simulink model "Copy_of_Model_vmaRHTS_R2019b"  (R2023a)
settings: Solver=ode4  StartTime=0.0  StopTime=tend  FixedStep=dt  RelTol=1e-3
undefined symbols (not defined in the file or in its folder): a0, a1, a2, a3, a4, a5, a6, a7, A_cplant, Ag, AgN, alpha1, alpha2, B_cplant, C_cplant, C_phys_5dof, CNrt, Continuous, CRrt, D_cplant, dt, dv1, dv2, EQ_intensity, EQ_sw, F, FN, K, K_1, K_2, K_phys_5dof, Kbar_inv, KI, KI_1, KI_2, KNbar_inv, Koo, Kot, l, lN, M_phys_5dof, MNrt, MRrt, Rbar, RNbar, Seed_snr, Time
libraries: simulink x6, slpidlib x4, ctrlSharedLib x3, sldrtlib x1
(part 1 of 3)
settings Model: Creator=icu327  LastModifiedBy=liangyu
settings SolverCC: AlgebraicLoopSolver=TrustRegion
settings DataIOCC: SaveFormat=Array  ReturnWorkspaceOutputs=off
settings DebuggingCC: UnconnectedInputMsg=warning  UnconnectedOutputMsg=warning  UnconnectedLineMsg=warning  ArithmeticOperatorsInVariantConditions=warning
settings HardwareCC: ProdBitPerLong=64  ProdHWDeviceType=Intel->x86-64 (Linux 64)
settings ModelReferenceCC: EnableRefExpFcnMdlSchedulingChecks=on
settings SFSimCC: CustomCodeUndefinedFunction=UseInterfaceOnly
settings RTWCC: Description=Simulink Desktop Real-Time  SystemTargetFile=sldrt.tlc  TemplateMakefile=sldrt.tmf  RTWCompilerOptimization=on
settings CodeAppCC: MaxIdLength=95  StateflowObjectComments=on
settings SimulinkDesktopRealTimeCC: TargetLibSuffix=_sldrt.a  TargetPreCompLibLocation=C:\Program Files\MATLAB\R2023a\toolbox\sldrt\lib\win64

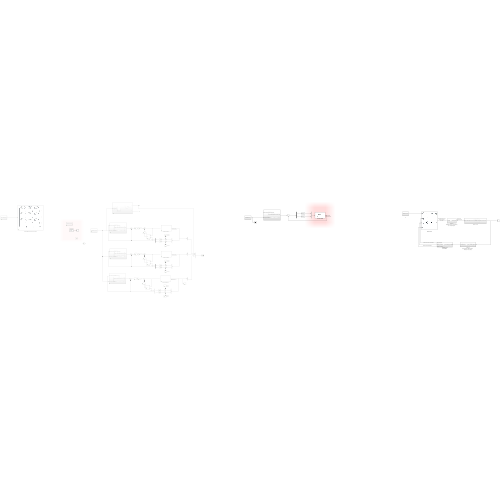
[thumbnail: Simulink's stored preview of the top-level diagram]
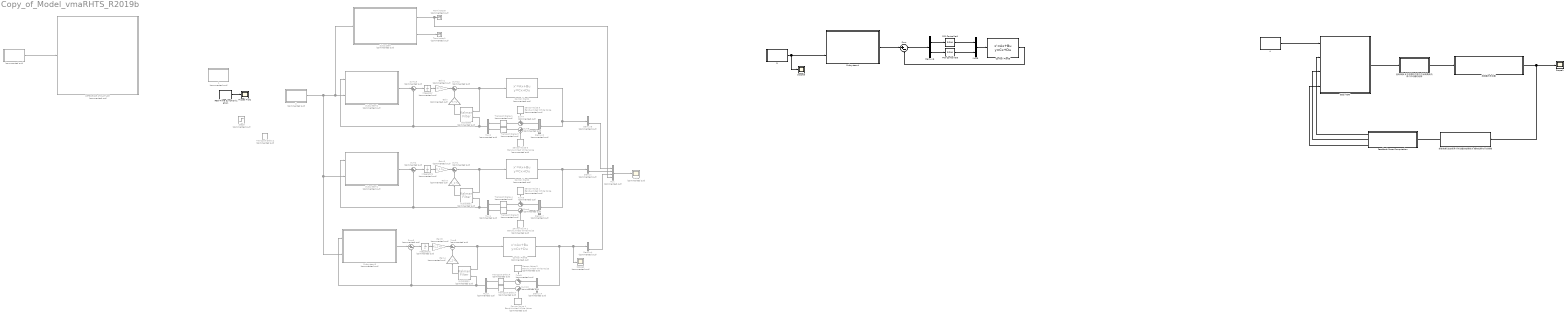
== system Copy_of_Model_vmaRHTS_R2019b ==
  " " : Subsystem  Commented=on
  " 1" : Subsystem  Commented=on
  " 2" : Subsystem  Commented=on
  " 3" : Subsystem
  " 4" : Subsystem
  " REFERENCE STRUCTURE" : Subsystem  Commented=on
      mask Display: image('$imagefile'); % Use "Edit Image" on toolstrip to change.
  " 数值子结构" : Subsystem
      mask Display: image('$imagefile'); % Use "Edit Image" on toolstrip to change.
  Control Plant1 : StateSpace  Commented=on  A=A_cplant  B=B_cplant  C=C_cplant  D=D_cplant  InitialCondition=0
  Control Plant2 : StateSpace  Commented=on  A=A_cplant  B=B_cplant  C=C_cplant  D=D_cplant  InitialCondition=0
  Control Plant3 : StateSpace  Commented=on  A=A_cplant  B=B_cplant  C=C_cplant  D=D_cplant  InitialCondition=0
  Control Plant5 : StateSpace  A=A_cplant  B=B_cplant  C=C_cplant  D=D_cplant  InitialCondition=0
  Demux{,1..5} (6 alike) : Demux  Commented=on  Outputs=2
  Demux6 : Demux  Outputs=2
  Feedback Force Computation : Subsystem
  Gain : Gain  Commented=on  Gain=K  Multiplication=Matrix(K*u) (u vector)
  Gain1 : Gain  Commented=on  Gain=KI  Multiplication=Matrix(K*u) (u vector)
  Gain2 : Gain  Commented=on  Gain=K_1  Multiplication=Matrix(K*u) (u vector)
  Gain3 : Gain  Commented=on  Gain=KI_1  Multiplication=Matrix(K*u) (u vector)
  Gain4 : Gain  Commented=on  Gain=K_2  Multiplication=Matrix(K*u) (u vector)
  Gain5 : Gain  Commented=on  Gain=KI_2  Multiplication=Matrix(K*u) (u vector)
  Integrator : Integrator  Commented=on
  Integrator1 : Integrator  Commented=on
  Integrator2 : Integrator  Commented=on
  Missed Ticks : Scope
  Mux : Mux  Commented=on
  Mux1 : Mux  Commented=on  Inputs=2
  Mux2 : Mux  Commented=on  Inputs=2
  Mux3 : Mux  Commented=on  Inputs=2
  Mux5 : Mux  Inputs=2
  PID Controller1 : slpidlib/PID Controller  Controller=PID  Form=Parallel  TimeDomain=Discrete-time  UseExternalTs=off  SampleTime=-1  IntegratorMethod=Forward Euler  FilterMethod=Forward Euler  ControllerParametersSource=internal  P=1  I=50  UseKiTs=off  D=1e-10  N=100  UseFilter=off  TunerSelectOption=Transfer Function Based (PID Tuner App)  InitialConditionSource=internal  InitialConditionForIntegrator=0  InitialConditionForFilter=0  DifferentiatorICPrevScaledInput=0  ExternalReset=none  TrackingMode=off  Kt=1  LimitOutput=off  SatLimitsSource=internal  UpperSaturationLimit=inf  LowerSaturationLimit=-inf  LinearizeAsGain=on  AntiWindupMode=none  Kb=1  LimitIntegrator=off  UpperIntegratorSaturationLimit=inf  LowerIntegratorSaturationLimit=-inf  POutMin=[]  POutMax=[]  IOutMin=[]  IOutMax=[]  DOutMin=[]  DOutMax=[]  NOutMin=[]  NOutMax=[]  SumOutMin=[]  SumOutMax=[]  SaturationOutMin=[]  SaturationOutMax=[]  PParamMin=[]  PParamMax=[]  IParamMin=[]  IParamMax=[]  DParamMin=[]  DParamMax=[]  NParamMin=[]  NParamMax=[]  KbParamMin=[]  KbParamMax=[]  KtParamMin=[]  KtParamMax=[]  KbOutMin=[]  KbOutMax=[]  KtOutMin=[]  KtOutMax=[]  IntegratorOutMin=[]  IntegratorOutMax=[]  FilterOutMin=[]  FilterOutMax=[]  SumI1OutMin=[]  SumI1OutMax=[]  SumI2OutMin=[]  SumI2OutMax=[]  SumI3OutMin=[]  SumI3OutMax=[]  SumI4OutMin=[]  SumI4OutMax=[]  SumDOutMin=[]  SumDOutMax=[]  DifferentiatorOutMin=[]  DifferentiatorOutMax=[]  FilterDiffOutCoefMin=[]  FilterDiffOutCoefMax=[]  ReciprocalOutMin=[]  ReciprocalOutMax=[]  SumDenOutMin=[]  SumDenOutMax=[]  SumNumOutMin=[]  SumNumOutMax=[]  DivideOutMin=[]  DivideOutMax=[]  UdiffTsProdOutMin=[]  UdiffTsProdOutMax=[]  NTsProdOutMin=[]  NTsProdOutMax=[]  UintegralTsProdOutMin=[]  UintegralTsProdOutMax=[]  UngainTsProdOutMin=[]  UngainTsProdOutMax=[]  ClampingZeroOutDataTypeStr=Inherit: Inherit via back propagation  ClampingZeroOutMin=[]  ClampingZeroOutMax=[]  FilterDenConstantOutDataTypeStr=Inherit: Inherit via back propagation  FilterDenConstantOutMin=[]  FilterDenConstantOutMax=[]  PCopyOutDataTypeStr=Inherit: Inherit via back propagation  PCopyOutMin=[]  PCopyOutMax=[]  NCopyOutDataTypeStr=Inherit: Inherit via back propagation  NCopyOutMin=[]  NCopyOutMax=[]  IntegratorContinuousStateAttributes=''  IntegratorStateMustResolveToSignalObject=off  IntegratorRTWStateStorageClass=Auto  FilterContinuousStateAttributes=''  FilterStateMustResolveToSignalObject=off  FilterRTWStateStorageClass=Auto  ParallelPVariant=InternalParameters  IdealPVariant=Disabled  IVariant=InternalParameters  DVariant=InternalParameters  IntegratorVariant=Discrete  SatVariant=Disabled  AWVariant=Passthrough  PCopyVariant=Disabled  TRVariant=Disabled  FdbkBlocksVariant=Forward  IdealPFdbkVariant=Disabled  SatFdbkVariant=Disabled  DerivativeFilterVariant=Differentiator  NVariant=Passthrough  NCopyVariant=Disabled_SignalSpec  FilterICVariant=InternalICsDifferentiator  IntegratorICVariant=InternalICs  ExternalResetVariant=Disabled  TRSumVariant=Passthrough  SumFdbkVariant=Disabled  SumVariant=Sum_PID  TsampFilterVariant=InternalTs  TsampNgainVariant=Passthrough  TsampIntegralVariant=Disabled_SignalSpec  ExternalSaturationOutDataTypeStr=Inherit: Same as second input
  PID Controller3 : slpidlib/PID Controller  Controller=PID  Form=Parallel  TimeDomain=Discrete-time  UseExternalTs=off  SampleTime=-1  IntegratorMethod=Forward Euler  FilterMethod=Forward Euler  ControllerParametersSource=internal  P=1  I=50  UseKiTs=off  D=1e-10  N=100  UseFilter=on  TunerSelectOption=Transfer Function Based (PID Tuner App)  InitialConditionSource=internal  InitialConditionForIntegrator=0  InitialConditionForFilter=0  DifferentiatorICPrevScaledInput=0  ExternalReset=none  TrackingMode=off  Kt=1  LimitOutput=off  SatLimitsSource=internal  UpperSaturationLimit=inf  LowerSaturationLimit=-inf  LinearizeAsGain=on  AntiWindupMode=none  Kb=1  LimitIntegrator=off  UpperIntegratorSaturationLimit=inf  LowerIntegratorSaturationLimit=-inf  POutMin=[]  POutMax=[]  IOutMin=[]  IOutMax=[]  DOutMin=[]  DOutMax=[]  NOutMin=[]  NOutMax=[]  SumOutMin=[]  SumOutMax=[]  SaturationOutMin=[]  SaturationOutMax=[]  PParamMin=[]  PParamMax=[]  IParamMin=[]  IParamMax=[]  DParamMin=[]  DParamMax=[]  NParamMin=[]  NParamMax=[]  KbParamMin=[]  KbParamMax=[]  KtParamMin=[]  KtParamMax=[]  KbOutMin=[]  KbOutMax=[]  KtOutMin=[]  KtOutMax=[]  IntegratorOutMin=[]  IntegratorOutMax=[]  FilterOutMin=[]  FilterOutMax=[]  SumI1OutMin=[]  SumI1OutMax=[]  SumI2OutMin=[]  SumI2OutMax=[]  SumI3OutMin=[]  SumI3OutMax=[]  SumI4OutMin=[]  SumI4OutMax=[]  SumDOutMin=[]  SumDOutMax=[]  DifferentiatorOutMin=[]  DifferentiatorOutMax=[]  FilterDiffOutCoefMin=[]  FilterDiffOutCoefMax=[]  ReciprocalOutMin=[]  ReciprocalOutMax=[]  SumDenOutMin=[]  SumDenOutMax=[]  SumNumOutMin=[]  SumNumOutMax=[]  DivideOutMin=[]  DivideOutMax=[]  UdiffTsProdOutMin=[]  UdiffTsProdOutMax=[]  NTsProdOutMin=[]  NTsProdOutMax=[]  UintegralTsProdOutMin=[]  UintegralTsProdOutMax=[]  UngainTsProdOutMin=[]  UngainTsProdOutMax=[]  ClampingZeroOutDataTypeStr=Inherit: Inherit via back propagation  ClampingZeroOutMin=[]  ClampingZeroOutMax=[]  FilterDenConstantOutDataTypeStr=Inherit: Inherit via back propagation  FilterDenConstantOutMin=[]  FilterDenConstantOutMax=[]  PCopyOutDataTypeStr=Inherit: Inherit via back propagation  PCopyOutMin=[]  PCopyOutMax=[]  NCopyOutDataTypeStr=Inherit: Inherit via back propagation  NCopyOutMin=[]  NCopyOutMax=[]  IntegratorContinuousStateAttributes=''  IntegratorStateMustResolveToSignalObject=off  IntegratorRTWStateStorageClass=Auto  FilterContinuousStateAttributes=''  FilterStateMustResolveToSignalObject=off  FilterRTWStateStorageClass=Auto  ParallelPVariant=InternalParameters  IdealPVariant=Disabled  IVariant=InternalParameters  DVariant=InternalParameters  IntegratorVariant=Discrete  SatVariant=Disabled  AWVariant=Passthrough  PCopyVariant=Disabled  TRVariant=Disabled  FdbkBlocksVariant=Forward  IdealPFdbkVariant=Disabled  SatFdbkVariant=Disabled  DerivativeFilterVariant=ForwardEulerFilter  NVariant=InternalParameters  NCopyVariant=Disabled  FilterICVariant=InternalICsFilter  IntegratorICVariant=InternalICs  ExternalResetVariant=Disabled  TRSumVariant=Passthrough  SumFdbkVariant=Disabled  SumVariant=Sum_PID  TsampFilterVariant=InternalTs  TsampNgainVariant=Passthrough  TsampIntegralVariant=Disabled_SignalSpec  ExternalSaturationOutDataTypeStr=Inherit: Same as second input
  Real-Time Synchronization : sldrtlib/Real-Time Synchronization  SampleTime=dt  MaxMissedTicks=10000  ShowMissedTicks=on  YieldWhenWaiting=off
  Scope : Scope  Commented=on
  Scope1 : Scope
  Scope2 : Scope  Commented=on
  Scope3 : Scope
  Sensor Noise {1..6} (6 alike) : simulink/Sources/Band-Limited White Noise  Commented=on  Cov=rms_noise_DT  Ts=dt  seed=double(Seed_snr.Seed)
  Step5 : Step  Commented=on  SampleTime=0
  Subsystem : Subsystem  Commented=on
  Subsystem1 : Subsystem  Commented=on
  Subsystem2 : Subsystem  Commented=on
  Subsystem3 : Subsystem  Commented=on
  Subsystem4 : Subsystem
  Sum : Sum  Inputs=|+-
  Sum{1..2,5..6,12..13} (6 alike) : Sum  Commented=on  Inputs=|+-
  Sum10 : Sum  Commented=on  Inputs=|++
  Sum3 : Sum  Commented=on  Inputs=++|
  Sum4 : Sum  Commented=on  Inputs=|++
  Sum7 : Sum  Commented=on  Inputs=++|
  Sum8 : Sum  Commented=on  Inputs=|++
  Sum9 : Sum  Commented=on  Inputs=++|
  Terminator1 : Terminator  Commented=on
  Terminator5 : Terminator  Commented=on
  Transport Delay1 : TransportDelay  Commented=on  DelayTime=0.04
  Transport Delay{2,4..7} (5 alike) : TransportDelay  Commented=on  DelayTime=0.03
  Transport Delay3 : TransportDelay  Commented=on  DelayTime=0.07
  "坐标转换 此处将两个作动器的位移转为 横向位移与节点转角 " : Subsystem
  坐标转换 此处将横向位移与节点转角转为 两个作动器的位移 : Subsystem
  控制器与作动器 : Subsystem
  状态观测器 : ctrlSharedLib/Kalman Filter  Commented=on  TimeDomain=Continuous-Time  UseCurrentEstimator=on  ModelSource=Individual A, B, C, D matrices  ModelSourceVariable=ss(0.95,1,1,0,1)  A=A_cplant  B=B_cplant  C=C_cplant  D=D_cplant  NumberOfStates=1  NumberOfInputs=1  NumberOfOutputs=1  InitialEstimateSource=Dialog  X0=0  P0=10  UseK=off  UseGH=off  NumberOfProcessNoiseInputs=1  G=1  TimeInvariantG=on  H=0  TimeInvariantH=on  Q=0.01*diag([1,1,1,1,1,1,1,1])  TimeInvariantQ=on  R=diag([1,1])  TimeInvariantR=on  N=0  TimeInvariantN=on  AddInputPort=on  AddEnablePort=off  OutputEstimatedY=off  OutputP=off  Ts=-1
  状态观测器1 : ctrlSharedLib/Kalman Filter  Commented=on  TimeDomain=Continuous-Time  UseCurrentEstimator=on  ModelSource=Individual A, B, C, D matrices  ModelSourceVariable=ss(0.95,1,1,0,1)  A=A_cplant  B=B_cplant  C=C_cplant  D=D_cplant  NumberOfStates=1  NumberOfInputs=1  NumberOfOutputs=1  InitialEstimateSource=Dialog  X0=0  P0=10  UseK=off  UseGH=off  NumberOfProcessNoiseInputs=1  G=1  TimeInvariantG=on  H=0  TimeInvariantH=on  Q=0.01*diag([1,1,1,1,1,1,1,1])  TimeInvariantQ=on  R=diag([1,1])  TimeInvariantR=on  N=0  TimeInvariantN=on  AddInputPort=on  AddEnablePort=off  OutputEstimatedY=off  OutputP=off  Ts=-1
  状态观测器2 : ctrlSharedLib/Kalman Filter  Commented=on  TimeDomain=Continuous-Time  UseCurrentEstimator=on  ModelSource=Individual A, B, C, D matrices  ModelSourceVariable=ss(0.95,1,1,0,1)  A=A_cplant  B=B_cplant  C=C_cplant  D=D_cplant  NumberOfStates=1  NumberOfInputs=1  NumberOfOutputs=1  InitialEstimateSource=Dialog  X0=0  P0=10  UseK=off  UseGH=off  NumberOfProcessNoiseInputs=1  G=1  TimeInvariantG=on  H=0  TimeInvariantH=on  Q=0.01*diag([1,1,1,1,1,1,1,1])  TimeInvariantQ=on  R=diag([1,1])  TimeInvariantR=on  N=0  TimeInvariantN=on  AddInputPort=on  AddEnablePort=off  OutputEstimatedY=off  OutputP=off  Ts=-1
  wires:
  " "/1(GROUND ACCEL) -> " REFERENCE STRUCTURE"/1(Ground_Acceleration)
  Real-Time Synchronization/1 -> Missed Ticks/1
  Mux2/1 -> 状态观测器/2, Subsystem2/1(Filtered actuator displacement vector), Sum13/2  "[u1,u2] (mm)"
  Sum7/1 -> Transport Delay1/1
  Sum8/1 -> Transport Delay3/1
  Sensor Noise 5/1 -> Sum7/1
  Subsystem2/1(Target actuator displacement vector (mm)) -> Sum13/1
  Control Plant1/1 -> Demux2/1, Demux5/1  "Filtered actuator displacement vector"
  Demux2/1 -> Sum7/2
  Sensor Noise 6/1 -> Sum8/2
  Demux2/2 -> Sum8/1
  Sum12/1 -> Control Plant1/1, 状态观测器/1
  状态观测器/1 -> Gain/1
  Gain/1 -> Sum12/2
  Sum13/1 -> Integrator/1
  Gain1/1 -> Sum12/1
  Integrator/1 -> Gain1/1
  Demux1/1 -> Sum3/2
  Gain3/1 -> Sum1/1
  Sum1/1 -> Control Plant2/1, 状态观测器1/1
  Mux1/1 -> 状态观测器1/2, Subsystem1/1(Filtered actuator displacement vector), Sum2/2  "[u1,u2] (mm)"
  Sum2/1 -> Integrator1/1
  Gain2/1 -> Sum1/2
  状态观测器1/1 -> Gain2/1
  Sensor Noise 1/1 -> Sum3/1
  Subsystem1/1(Target actuator displacement vector (mm)) -> Sum2/1
  Control Plant2/1 -> Demux/1, Demux1/1  "Filtered actuator displacement vector"
  Sensor Noise 2/1 -> Sum4/2
  Demux1/2 -> Sum4/1
  Integrator1/1 -> Gain3/1
  Sum3/1 -> Transport Delay4/1
  Sum4/1 -> Transport Delay5/1
  Demux3/1 -> Sum9/2
  Gain5/1 -> Sum5/1
  Sum5/1 -> Control Plant3/1, 状态观测器2/1
  Mux3/1 -> 状态观测器2/2, Subsystem3/1(Filtered actuator displacement vector), Sum6/2  "[u1,u2] (mm)"
  Sum6/1 -> Integrator2/1
  Gain4/1 -> Sum5/2
  状态观测器2/1 -> Gain4/1
  Sensor Noise 3/1 -> Sum9/1
  Subsystem3/1(Target actuator displacement vector (mm)) -> Sum6/1
  Control Plant3/1 -> Scope2/1, Demux4/1, Demux3/1  "Filtered actuator displacement vector"
  Sensor Noise 4/1 -> Sum10/2
  Demux3/2 -> Sum10/1
  Integrator2/1 -> Gain5/1
  Sum9/1 -> Transport Delay6/1
  Sum10/1 -> Transport Delay7/1
  Mux/1 -> Scope/1
  Demux/2 -> Mux/2
  Demux4/2 -> Mux/3
  " 2"/1(GROUND ACCEL) -> Subsystem/1(accel_grd), Subsystem2/2(Ground_Acceleration), Subsystem3/2(Ground_Acceleration), Subsystem1/2(Ground_Acceleration)
  Subsystem/1(Out1) -> Mux/4, Terminator5/1
  Subsystem/2(Out2) -> Terminator1/1
  Demux5/2 -> Mux/1
  Transport Delay1/1 -> Mux2/1
  Transport Delay3/1 -> Mux2/2
  Transport Delay4/1 -> Mux1/1
  Transport Delay5/1 -> Mux1/2
  Transport Delay6/1 -> Mux3/1
  Transport Delay7/1 -> Mux3/2
  " 3"/1(GROUND ACCEL) -> Scope3/1, Subsystem4/2(Ground_Acceleration)
  Demux6/1 -> PID Controller1/1
  Demux6/2 -> PID Controller3/1
  Mux5/1 -> Control Plant5/1
  Subsystem4/1(Target actuator displacement vector (mm)) -> Sum/1
  Sum/1 -> Demux6/1
  PID Controller1/1 -> Mux5/1
  PID Controller3/1 -> Mux5/2
  Feedback Force Computation/1(F(27)_phys (N)) -> " 数值子结构"/2(RTHS_feedback_Force27)  "Feedback Force at Controlled Node"
  Feedback Force Computation/3(M(29)_phys (N*m)) -> " 数值子结构"/4(RTHS_feedback_Moment29)  "Moment at Uncontrolled Node"
  "坐标转换 此处将两个作动器的位移转为 横向位移与节点转角 "/1("[x, theta] (m, rad)") -> Feedback Force Computation/1("[x_est, theta_est] (m,rad)")
  " 数值子结构"/1(Linear Displacement 27) -> 坐标转换 此处将横向位移与节点转角转为 两个作动器的位移/1("[x, theta]")  "Target displacement vector Frame coordinates (mm, rad)"
  " 4"/1(GROUND ACCEL) -> " 数值子结构"/1(Ground_Acceleration)
  Feedback Force Computation/2(M(21)_phys (N*m)) -> " 数值子结构"/3(RTHS_feedback_Moment21)  "Moment at Controlled Node"
  Control Plant5/1 -> Sum/2  "Filtered actuator displacement vector"
  坐标转换 此处将横向位移与节点转角转为 两个作动器的位移/1("[xa1,xa2] mm") -> 控制器与作动器/1(Target actuator displacement vector (mm))  "Target actuator displacement vector (mm)"
  控制器与作动器/1(Filtered actuator displacement vector) -> Scope1/1, "坐标转换 此处将两个作动器的位移转为 横向位移与节点转角 "/1("[xm1_est, xm2_est] (mm)")

== system Copy_of_Model_vmaRHTS_R2019b/  ==
  note: Benchmark Control Problem for
      | Multi-axial Real-time Hybrid Simulation
      | Ground Acceleration
  Clock : Clock
  EQ scaling factor : Gain  Gain=EQ_intensity  Multiplication=Matrix(K*u)
  GROUND ACCELERATION : ToWorkspace  VariableName=EQ_input  SampleTime=-1
      settings: Save2DSignal=2-D array (concatenate along first dimension)
  Ground motion record : Subsystem
  Multiport Switch : MultiPortSwitch  SaturateOnIntegerOverflow=off  InputSameDT=off
  SWITCH CONSTANT : Constant  Value=EQ_sw
  To Workspace : ToWorkspace  VariableName=t  SampleTime=dt
  GROUND ACCEL : Outport  VectorParamsAs1DForOutWhenUnconnected=off
  wires:
  Multiport Switch/1 -> EQ scaling factor/1
  EQ scaling factor/1 -> GROUND ACCELERATION/1, GROUND ACCEL/1
  Ground motion record/1(El Centro) -> Multiport Switch/2
  Ground motion record/2(Kobe) -> Multiport Switch/3
  Ground motion record/3(Morgan) -> Multiport Switch/4
  SWITCH CONSTANT/1 -> Multiport Switch/1
  Clock/1 -> To Workspace/1

== system Copy_of_Model_vmaRHTS_R2019b/ 1 ==
  note: Benchmark Control Problem for
      | Multi-axial Real-time Hybrid Simulation
      | Ground Acceleration
  Clock : Clock
  EQ scaling factor : Gain  Gain=EQ_intensity  Multiplication=Matrix(K*u)
  GROUND ACCELERATION : ToWorkspace  VariableName=EQ_input  SampleTime=-1
      settings: Save2DSignal=2-D array (concatenate along first dimension)
  Ground motion record : Subsystem
  Multiport Switch : MultiPortSwitch  SaturateOnIntegerOverflow=off  InputSameDT=off
  SWITCH CONSTANT : Constant  Value=EQ_sw
  To Workspace : ToWorkspace  VariableName=t  SampleTime=dt
  GROUND ACCEL : Outport  VectorParamsAs1DForOutWhenUnconnected=off
  wires:
  Multiport Switch/1 -> EQ scaling factor/1
  EQ scaling factor/1 -> GROUND ACCELERATION/1, GROUND ACCEL/1
  Ground motion record/1(El Centro) -> Multiport Switch/2
  Ground motion record/2(Kobe) -> Multiport Switch/3
  Ground motion record/3(Morgan) -> Multiport Switch/4
  SWITCH CONSTANT/1 -> Multiport Switch/1
  Clock/1 -> To Workspace/1

== system Copy_of_Model_vmaRHTS_R2019b/ 2 ==
  note: Benchmark Control Problem for
      | Multi-axial Real-time Hybrid Simulation
      | Ground Acceleration
  Clock : Clock
  EQ scaling factor : Gain  Gain=EQ_intensity  Multiplication=Matrix(K*u)
  GROUND ACCELERATION : ToWorkspace  VariableName=EQ_input  SampleTime=-1
      settings: Save2DSignal=2-D array (concatenate along first dimension)
  Ground motion record : Subsystem
  Multiport Switch : MultiPortSwitch  SaturateOnIntegerOverflow=off  InputSameDT=off
  SWITCH CONSTANT : Constant  Value=EQ_sw
  To Workspace : ToWorkspace  VariableName=t  SampleTime=dt
  GROUND ACCEL : Outport  VectorParamsAs1DForOutWhenUnconnected=off
  wires:
  Multiport Switch/1 -> EQ scaling factor/1
  EQ scaling factor/1 -> GROUND ACCELERATION/1, GROUND ACCEL/1
  Ground motion record/1(El Centro) -> Multiport Switch/2
  Ground motion record/2(Kobe) -> Multiport Switch/3
  Ground motion record/3(Morgan) -> Multiport Switch/4
  SWITCH CONSTANT/1 -> Multiport Switch/1
  Clock/1 -> To Workspace/1

== system Copy_of_Model_vmaRHTS_R2019b/ 3 ==
  note: Benchmark Control Problem for
      | Multi-axial Real-time Hybrid Simulation
      | Ground Acceleration
  Clock : Clock
  EQ scaling factor : Gain  Gain=EQ_intensity  Multiplication=Matrix(K*u)
  GROUND ACCELERATION : ToWorkspace  VariableName=EQ_input  SampleTime=-1
      settings: Save2DSignal=2-D array (concatenate along first dimension)
  Ground motion record : Subsystem
  Multiport Switch : MultiPortSwitch  SaturateOnIntegerOverflow=off  InputSameDT=off
  SWITCH CONSTANT : Constant  Value=EQ_sw
  To Workspace : ToWorkspace  VariableName=t  SampleTime=dt
  GROUND ACCEL : Outport  VectorParamsAs1DForOutWhenUnconnected=off
  wires:
  Multiport Switch/1 -> EQ scaling factor/1
  EQ scaling factor/1 -> GROUND ACCELERATION/1, GROUND ACCEL/1
  Ground motion record/1(El Centro) -> Multiport Switch/2
  Ground motion record/2(Kobe) -> Multiport Switch/3
  Ground motion record/3(Morgan) -> Multiport Switch/4
  SWITCH CONSTANT/1 -> Multiport Switch/1
  Clock/1 -> To Workspace/1

== system Copy_of_Model_vmaRHTS_R2019b/ 4 ==
  note: Benchmark Control Problem for
      | Multi-axial Real-time Hybrid Simulation
      | Ground Acceleration
  Clock : Clock
  EQ scaling factor : Gain  Gain=EQ_intensity  Multiplication=Matrix(K*u)
  GROUND ACCELERATION : ToWorkspace  VariableName=EQ_input  SampleTime=-1
      settings: Save2DSignal=2-D array (concatenate along first dimension)
  Ground motion record : Subsystem
  Multiport Switch : MultiPortSwitch  SaturateOnIntegerOverflow=off  InputSameDT=off
  SWITCH CONSTANT : Constant  Value=EQ_sw
  To Workspace : ToWorkspace  VariableName=t  SampleTime=dt
  GROUND ACCEL : Outport  VectorParamsAs1DForOutWhenUnconnected=off
  wires:
  Multiport Switch/1 -> EQ scaling factor/1
  EQ scaling factor/1 -> GROUND ACCELERATION/1, GROUND ACCEL/1
  Ground motion record/1(El Centro) -> Multiport Switch/2
  Ground motion record/2(Kobe) -> Multiport Switch/3
  Ground motion record/3(Morgan) -> Multiport Switch/4
  SWITCH CONSTANT/1 -> Multiport Switch/1
  Clock/1 -> To Workspace/1

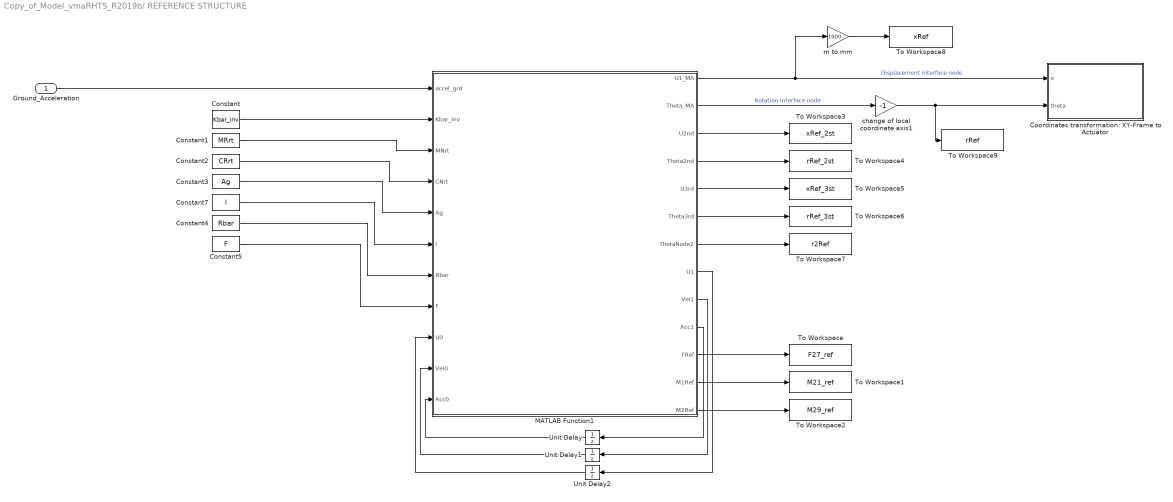
== system Copy_of_Model_vmaRHTS_R2019b/ REFERENCE STRUCTURE ==
  Ground_Acceleration : Inport
  Constant : Constant  Value=Kbar_inv  VectorParams1D=off
  Constant1 : Constant  Value=MRrt  VectorParams1D=off
  Constant2 : Constant  Value=CRrt  VectorParams1D=off
  Constant3 : Constant  Value=Ag  VectorParams1D=off
  Constant4 : Constant  Value=Rbar  VectorParams1D=off
  Constant5 : Constant  Value=F  VectorParams1D=off
  Constant7 : Constant  Value=l  VectorParams1D=off
  "Coordinates transformation: XY-Frame to Actuator " : Subsystem
  MATLAB Function1 : MATLAB Function  TreatAsAtomicUnit=on
  To Workspace : ToWorkspace  VariableName=F27_ref  SampleTime=-1
  To Workspace1 : ToWorkspace  VariableName=M21_ref  SampleTime=-1
  To Workspace2 : ToWorkspace  VariableName=M29_ref  SampleTime=-1
  To Workspace3 : ToWorkspace  VariableName=xRef_2st  SampleTime=dt
  To Workspace4 : ToWorkspace  VariableName=rRef_2st  SampleTime=dt
  To Workspace5 : ToWorkspace  VariableName=xRef_3st  SampleTime=dt
  To Workspace6 : ToWorkspace  VariableName=rRef_3st  SampleTime=dt
  To Workspace7 : ToWorkspace  VariableName=r2Ref  SampleTime=dt
  To Workspace8 : ToWorkspace  VariableName=xRef  SampleTime=dt
  To Workspace9 : ToWorkspace  VariableName=rRef  SampleTime=dt
  Unit Delay : UnitDelay  SampleTime=-1  HasFrameUpgradeWarning=on
  Unit Delay1 : UnitDelay  SampleTime=-1  HasFrameUpgradeWarning=on
  Unit Delay2 : UnitDelay  SampleTime=-1  HasFrameUpgradeWarning=on
  change of local coordinate axis1 : Gain  Gain=-1
  "m to mm  " : Gain  Gain=1000
  wires:
  Ground_Acceleration/1 -> MATLAB Function1/1(accel_grd)
  MATLAB Function1/1(U1_MA) -> "Coordinates transformation: XY-Frame to Actuator "/1(x), "m to mm  "/1  "Displacement interface node"
  MATLAB Function1/2(Theta_MA) -> change of local coordinate axis1/1  "Rotation interface node"
  Constant/1 -> MATLAB Function1/2(Kbar_inv)
  Constant1/1 -> MATLAB Function1/3(MNrt)
  Constant2/1 -> MATLAB Function1/4(CNrt)
  Constant3/1 -> MATLAB Function1/5(Ag)
  Constant7/1 -> MATLAB Function1/6(l)
  Constant4/1 -> MATLAB Function1/7(Rbar)
  Unit Delay2/1 -> MATLAB Function1/9(U0)
  Unit Delay1/1 -> MATLAB Function1/10(Vel0)
  Unit Delay/1 -> MATLAB Function1/11(Acc0)
  MATLAB Function1/9(Vel1) -> Unit Delay1/1
  MATLAB Function1/10(Acc1) -> Unit Delay/1
  MATLAB Function1/8(U1) -> Unit Delay2/1
  Constant5/1 -> MATLAB Function1/8(F)
  MATLAB Function1/13(M2Ref) -> To Workspace2/1
  MATLAB Function1/12(M1Ref) -> To Workspace1/1
  MATLAB Function1/11(FRef) -> To Workspace/1
  MATLAB Function1/3(U2nd) -> To Workspace3/1
  MATLAB Function1/4(Theta2nd) -> To Workspace4/1
  MATLAB Function1/5(U3rd) -> To Workspace5/1
  MATLAB Function1/6(Theta3rd) -> To Workspace6/1
  MATLAB Function1/7(ThetaNode2) -> To Workspace7/1
  "m to mm  "/1 -> To Workspace8/1
  change of local coordinate axis1/1 -> To Workspace9/1, "Coordinates transformation: XY-Frame to Actuator "/2(theta)

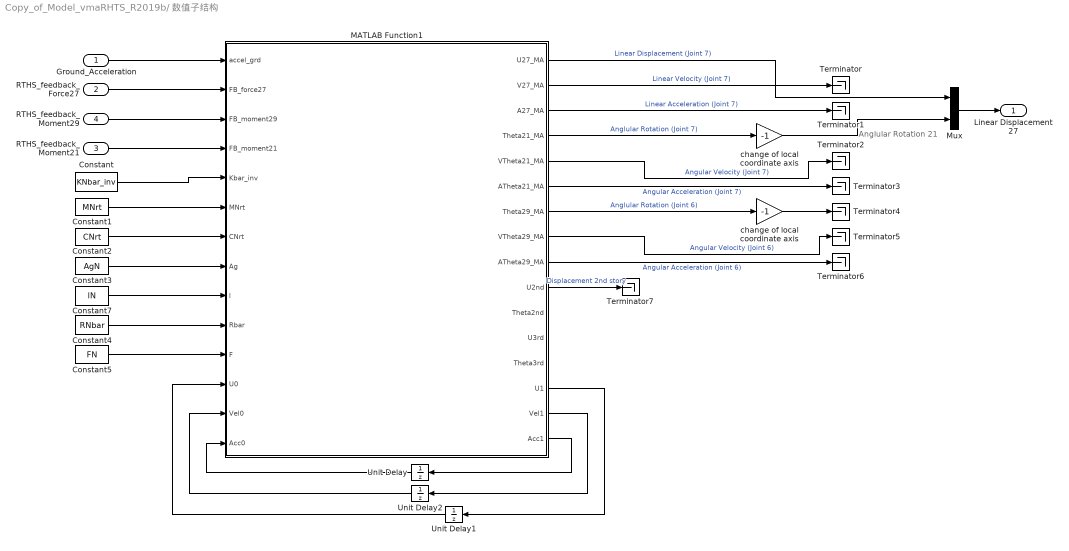
== system Copy_of_Model_vmaRHTS_R2019b/ 数值子结构 ==
  note: Anglular Rotation 21
  Ground_Acceleration : Inport
  RTHS_feedback_Force27 : Inport  Port=2
  RTHS_feedback_Moment21 : Inport  Port=3
  RTHS_feedback_Moment29 : Inport  Port=4
  Constant : Constant  Value=KNbar_inv  VectorParams1D=off
  Constant1 : Constant  Value=MNrt  VectorParams1D=off
  Constant2 : Constant  Value=CNrt  VectorParams1D=off
  Constant3 : Constant  Value=AgN  VectorParams1D=off
  Constant4 : Constant  Value=RNbar  VectorParams1D=off
  Constant5 : Constant  Value=FN  VectorParams1D=off
  Constant7 : Constant  Value=lN  VectorParams1D=off
  MATLAB Function1 : MATLAB Function  TreatAsAtomicUnit=on
  Mux : Mux  Inputs=2
  Terminator{,1..7} (8 alike) : Terminator
  Unit Delay : UnitDelay  SampleTime=-1  HasFrameUpgradeWarning=on
  Unit Delay1 : UnitDelay  SampleTime=-1  HasFrameUpgradeWarning=on
  Unit Delay2 : UnitDelay  SampleTime=-1  HasFrameUpgradeWarning=on
  change of local coordinate axis : Gain  Gain=-1
  "change of local coordinate axis  " : Gain  Gain=-1
  Linear Displacement 27 : Outport  VectorParamsAs1DForOutWhenUnconnected=off
  wires:
  Ground_Acceleration/1 -> MATLAB Function1/1(accel_grd)
  RTHS_feedback_Force27/1 -> MATLAB Function1/2(FB_force27)
  RTHS_feedback_Moment29/1 -> MATLAB Function1/3(FB_moment29)
  MATLAB Function1/1(U27_MA) -> Mux/1  "Linear Displacement (Joint 7)"
  MATLAB Function1/4(Theta21_MA) -> change of local coordinate axis/1  "Anglular Rotation (Joint 7)"
  Constant/1 -> MATLAB Function1/5(Kbar_inv)
  Constant1/1 -> MATLAB Function1/6(MNrt)
  Constant2/1 -> MATLAB Function1/7(CNrt)
  Constant3/1 -> MATLAB Function1/8(Ag)
  Constant7/1 -> MATLAB Function1/9(l)
  Constant4/1 -> MATLAB Function1/10(Rbar)
  Unit Delay1/1 -> MATLAB Function1/12(U0)
  Unit Delay2/1 -> MATLAB Function1/13(Vel0)
  Unit Delay/1 -> MATLAB Function1/14(Acc0)
  MATLAB Function1/15(Vel1) -> Unit Delay2/1
  MATLAB Function1/16(Acc1) -> Unit Delay/1
  MATLAB Function1/14(U1) -> Unit Delay1/1
  Constant5/1 -> MATLAB Function1/11(F)
  MATLAB Function1/2(V27_MA) -> Terminator/1  "Linear Velocity (Joint 7)"
  MATLAB Function1/3(A27_MA) -> Terminator1/1  "Linear Acceleration (Joint 7)"
  MATLAB Function1/5(VTheta21_MA) -> Terminator2/1  "Angular Velocity (Joint 7)"
  MATLAB Function1/6(ATheta21_MA) -> Terminator3/1  "Angular Acceleration (Joint 7)"
  MATLAB Function1/9(ATheta29_MA) -> Terminator6/1  "Angular Acceleration (Joint 6)"
  MATLAB Function1/8(VTheta29_MA) -> Terminator5/1  "Angular Velocity (Joint 6)"
  MATLAB Function1/7(Theta29_MA) -> "change of local coordinate axis  "/1  "Anglular Rotation (Joint 6)"
  RTHS_feedback_Moment21/1 -> MATLAB Function1/4(FB_moment21)
  change of local coordinate axis/1 -> Mux/2
  "change of local coordinate axis  "/1 -> Terminator4/1
  Mux/1 -> Linear Displacement 27/1
  MATLAB Function1/10(U2nd) -> Terminator7/1  "Displacement 2nd story"

== system Copy_of_Model_vmaRHTS_R2019b/Feedback Force Computation ==
  note: F(27)
  note: M(21)
  note: M(29)
  "[x_est, theta_est] (m,rad)" : Inport
  Demux : Demux  Outputs=3
  Derivative : Derivative
  Derivative1 : Derivative
  Gain : Gain  Gain=-inv(Koo)*Kot  Multiplication=Matrix(K*u) (u vector)
  Gain1 : Gain  Gain=K_phys_5dof  Multiplication=Matrix(K*u) (u vector)
  Gain2 : Gain  Gain=C_phys_5dof  Multiplication=Matrix(K*u) (u vector)
  Gain3 : Gain  Gain=M_phys_5dof  Multiplication=Matrix(K*u) (u vector)
  Mux1 : Mux  Inputs=2
  Selector : Selector  InputPortWidth=5  IndexOptions=Index vector (dialog)  Indices=[1 2 3]  OutputSizes=1
  Sum : Sum  Inputs=+|+|+
  change of local coordinate axis2 : Gain  Gain=-1
  change of local coordinate axis3 : Gain  Gain=-1
  F(27)_phys (N) : Outport  VectorParamsAs1DForOutWhenUnconnected=off
  M(21)_phys (N*m) : Outport  Port=2  VectorParamsAs1DForOutWhenUnconnected=off
  M(29)_phys (N*m) : Outport  Port=3  VectorParamsAs1DForOutWhenUnconnected=off
  wires:
  Gain/1 -> Mux1/2
  Derivative1/1 -> Gain3/1
  Gain2/1 -> Sum/2
  Derivative/1 -> Gain2/1, Derivative1/1
  Gain1/1 -> Sum/1
  "[x_est, theta_est] (m,rad)"/1 -> Gain/1, Mux1/1
  Demux/1 -> F(27)_phys (N)/1
  Sum/1 -> Selector/1
  Selector/1 -> Demux/1
  Gain3/1 -> Sum/3
  Demux/2 -> change of local coordinate axis2/1
  Demux/3 -> change of local coordinate axis3/1
  Mux1/1 -> Derivative/1, Gain1/1
  change of local coordinate axis2/1 -> M(21)_phys (N*m)/1
  change of local coordinate axis3/1 -> M(29)_phys (N*m)/1

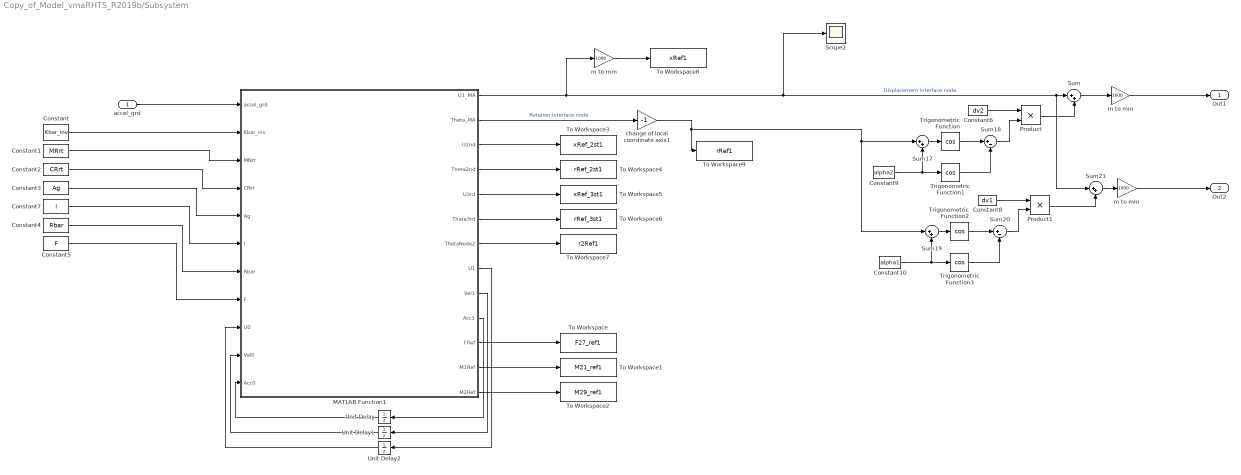
== system Copy_of_Model_vmaRHTS_R2019b/Subsystem ==
  accel_grd : Inport
  Constant : Constant  Value=Kbar_inv  VectorParams1D=off
  Constant1 : Constant  Value=MRrt  VectorParams1D=off
  Constant10 : Constant  Value=alpha1
  Constant2 : Constant  Value=CRrt  VectorParams1D=off
  Constant3 : Constant  Value=Ag  VectorParams1D=off
  Constant4 : Constant  Value=Rbar  VectorParams1D=off
  Constant5 : Constant  Value=F  VectorParams1D=off
  Constant6 : Constant  Value=dv2
  Constant7 : Constant  Value=l  VectorParams1D=off
  Constant8 : Constant  Value=dv1
  Constant9 : Constant  Value=alpha2
  MATLAB Function1 : MATLAB Function  TreatAsAtomicUnit=on
  Product : Product
  Product1 : Product
  Scope2 : Scope
  Sum{,17,19,21} (4 alike) : Sum  Inputs=|++
  Sum18 : Sum  Inputs=|+-
  Sum20 : Sum  Inputs=|+-
  To Workspace : ToWorkspace  VariableName=F27_ref1  SampleTime=-1
  To Workspace1 : ToWorkspace  VariableName=M21_ref1  SampleTime=-1
  To Workspace2 : ToWorkspace  VariableName=M29_ref1  SampleTime=-1
  To Workspace3 : ToWorkspace  VariableName=xRef_2st1  SampleTime=dt
  To Workspace4 : ToWorkspace  VariableName=rRef_2st1  SampleTime=dt
  To Workspace5 : ToWorkspace  VariableName=xRef_3st1  SampleTime=dt
  To Workspace6 : ToWorkspace  VariableName=rRef_3st1  SampleTime=dt
  To Workspace7 : ToWorkspace  VariableName=r2Ref1  SampleTime=dt
  To Workspace8 : ToWorkspace  VariableName=xRef1  SampleTime=dt
  To Workspace9 : ToWorkspace  VariableName=rRef1  SampleTime=dt
  Trigonometric Function{,1..3} (4 alike) : Trigonometry  Operator=cos
  Unit Delay : UnitDelay  SampleTime=-1  HasFrameUpgradeWarning=on
  Unit Delay1 : UnitDelay  SampleTime=-1  HasFrameUpgradeWarning=on
  Unit Delay2 : UnitDelay  SampleTime=-1  HasFrameUpgradeWarning=on
  change of local coordinate axis1 : Gain  Gain=-1
  m to mm : Gain  Gain=1000
  "m to mm " : Gain  Gain=1000
  "m to mm  " : Gain  Gain=1000
  Out1 : Outport
  Out2 : Outport  Port=2
  wires:
  MATLAB Function1/11(FRef) -> To Workspace/1
  "m to mm  "/1 -> To Workspace8/1
  MATLAB Function1/13(M2Ref) -> To Workspace2/1
  Sum18/1 -> Product/2
  Trigonometric Function1/1 -> Sum18/2
  MATLAB Function1/7(ThetaNode2) -> To Workspace7/1
  MATLAB Function1/5(U3rd) -> To Workspace5/1
  MATLAB Function1/4(Theta2nd) -> To Workspace4/1
  MATLAB Function1/1(U1_MA) -> "m to mm  "/1, Sum/1, Sum21/1, Scope2/1  "Displacement interface node"
  MATLAB Function1/8(U1) -> Unit Delay2/1
  Constant2/1 -> MATLAB Function1/4(CNrt)
  change of local coordinate axis1/1 -> Sum17/1, Sum19/1, To Workspace9/1
  Constant6/1 -> Product/1
  Unit Delay2/1 -> MATLAB Function1/9(U0)
  Constant9/1 -> Trigonometric Function1/1, Sum17/2
  MATLAB Function1/12(M1Ref) -> To Workspace1/1
  Constant8/1 -> Product1/1
  Constant10/1 -> Trigonometric Function3/1, Sum19/2
  Product/1 -> Sum/2
  Constant5/1 -> MATLAB Function1/8(F)
  Sum/1 -> m to mm/1
  Sum19/1 -> Trigonometric Function2/1
  Product1/1 -> Sum21/2
  Trigonometric Function2/1 -> Sum20/1
  MATLAB Function1/6(Theta3rd) -> To Workspace6/1
  Sum20/1 -> Product1/2
  Trigonometric Function/1 -> Sum18/1
  Sum17/1 -> Trigonometric Function/1
  Sum21/1 -> "m to mm "/1
  MATLAB Function1/2(Theta_MA) -> change of local coordinate axis1/1  "Rotation interface node"
  MATLAB Function1/9(Vel1) -> Unit Delay1/1
  Constant7/1 -> MATLAB Function1/6(l)
  Trigonometric Function3/1 -> Sum20/2
  Constant4/1 -> MATLAB Function1/7(Rbar)
  accel_grd/1 -> MATLAB Function1/1(accel_grd)
  Constant/1 -> MATLAB Function1/2(Kbar_inv)
  Unit Delay/1 -> MATLAB Function1/11(Acc0)
  m to mm/1 -> Out1/1
  Constant3/1 -> MATLAB Function1/5(Ag)
  Unit Delay1/1 -> MATLAB Function1/10(Vel0)
  Constant1/1 -> MATLAB Function1/3(MNrt)
  MATLAB Function1/3(U2nd) -> To Workspace3/1
  MATLAB Function1/10(Acc1) -> Unit Delay/1
  "m to mm "/1 -> Out2/1

== system Copy_of_Model_vmaRHTS_R2019b/Subsystem1 ==
  Filtered actuator displacement vector : Inport
  Ground_Acceleration : Inport  Port=2
  " NUMERICAL SUBSTRUCTURE" : Subsystem
      mask Display: image('$imagefile'); % Use "Edit Image" on toolstrip to change.
  Coordinate transformation: Actuator to Frame : Subsystem
  Coordinate transformation: Frame to Actuator : Subsystem
  Feedback Force Computation : Subsystem
  Target actuator displacement vector (mm) : Outport
  wires:
  Coordinate transformation: Actuator to Frame/1("[x, theta] (m, rad)") -> Feedback Force Computation/1("[x_est, theta_est] (m,rad)")
  Filtered actuator displacement vector/1 -> Coordinate transformation: Actuator to Frame/1("[xm1_est, xm2_est] (mm)")
  Feedback Force Computation/3(M(29)_phys (N*m)) -> " NUMERICAL SUBSTRUCTURE"/4(RTHS_feedback_Moment29)  "Moment at Uncontrolled Node"
  " NUMERICAL SUBSTRUCTURE"/1(Linear Displacement 27) -> Coordinate transformation: Frame to Actuator/1("[x, theta]")  "Target displacement vector Frame coordinates (mm, rad)"
  Feedback Force Computation/2(M(21)_phys (N*m)) -> " NUMERICAL SUBSTRUCTURE"/3(RTHS_feedback_Moment21)  "Moment at Controlled Node"
  Feedback Force Computation/1(F(27)_phys (N)) -> " NUMERICAL SUBSTRUCTURE"/2(RTHS_feedback_Force27)  "Feedback Force at Controlled Node"
  Ground_Acceleration/1 -> " NUMERICAL SUBSTRUCTURE"/1(Ground_Acceleration)
  Coordinate transformation: Frame to Actuator/1("[xa1,xa2] mm") -> Target actuator displacement vector (mm)/1  "Target actuator displacement vector (mm)"

== system Copy_of_Model_vmaRHTS_R2019b/Subsystem2 ==
  Filtered actuator displacement vector : Inport
  Ground_Acceleration : Inport  Port=2
  " NUMERICAL SUBSTRUCTURE" : Subsystem
      mask Display: image('$imagefile'); % Use "Edit Image" on toolstrip to change.
  Coordinate transformation: Actuator to Frame : Subsystem
  Coordinate transformation: Frame to Actuator : Subsystem
  Feedback Force Computation : Subsystem
  Target actuator displacement vector (mm) : Outport
  wires:
  Coordinate transformation: Actuator to Frame/1("[x, theta] (m, rad)") -> Feedback Force Computation/1("[x_est, theta_est] (m,rad)")
  Filtered actuator displacement vector/1 -> Coordinate transformation: Actuator to Frame/1("[xm1_est, xm2_est] (mm)")
  Feedback Force Computation/3(M(29)_phys (N*m)) -> " NUMERICAL SUBSTRUCTURE"/4(RTHS_feedback_Moment29)  "Moment at Uncontrolled Node"
  " NUMERICAL SUBSTRUCTURE"/1(Linear Displacement 27) -> Coordinate transformation: Frame to Actuator/1("[x, theta]")  "Target displacement vector Frame coordinates (mm, rad)"
  Feedback Force Computation/2(M(21)_phys (N*m)) -> " NUMERICAL SUBSTRUCTURE"/3(RTHS_feedback_Moment21)  "Moment at Controlled Node"
  Feedback Force Computation/1(F(27)_phys (N)) -> " NUMERICAL SUBSTRUCTURE"/2(RTHS_feedback_Force27)  "Feedback Force at Controlled Node"
  Ground_Acceleration/1 -> " NUMERICAL SUBSTRUCTURE"/1(Ground_Acceleration)
  Coordinate transformation: Frame to Actuator/1("[xa1,xa2] mm") -> Target actuator displacement vector (mm)/1  "Target actuator displacement vector (mm)"

== system Copy_of_Model_vmaRHTS_R2019b/Subsystem3 ==
  Filtered actuator displacement vector : Inport
  Ground_Acceleration : Inport  Port=2
  " NUMERICAL SUBSTRUCTURE" : Subsystem
      mask Display: image('$imagefile'); % Use "Edit Image" on toolstrip to change.
  Coordinate transformation: Actuator to Frame : Subsystem
  Coordinate transformation: Frame to Actuator : Subsystem
  Feedback Force Computation : Subsystem
  Target actuator displacement vector (mm) : Outport
  wires:
  Coordinate transformation: Actuator to Frame/1("[x, theta] (m, rad)") -> Feedback Force Computation/1("[x_est, theta_est] (m,rad)")
  Filtered actuator displacement vector/1 -> Coordinate transformation: Actuator to Frame/1("[xm1_est, xm2_est] (mm)")
  Feedback Force Computation/3(M(29)_phys (N*m)) -> " NUMERICAL SUBSTRUCTURE"/4(RTHS_feedback_Moment29)  "Moment at Uncontrolled Node"
  " NUMERICAL SUBSTRUCTURE"/1(Linear Displacement 27) -> Coordinate transformation: Frame to Actuator/1("[x, theta]")  "Target displacement vector Frame coordinates (mm, rad)"
  Feedback Force Computation/2(M(21)_phys (N*m)) -> " NUMERICAL SUBSTRUCTURE"/3(RTHS_feedback_Moment21)  "Moment at Controlled Node"
  Feedback Force Computation/1(F(27)_phys (N)) -> " NUMERICAL SUBSTRUCTURE"/2(RTHS_feedback_Force27)  "Feedback Force at Controlled Node"
  Ground_Acceleration/1 -> " NUMERICAL SUBSTRUCTURE"/1(Ground_Acceleration)
  Coordinate transformation: Frame to Actuator/1("[xa1,xa2] mm") -> Target actuator displacement vector (mm)/1  "Target actuator displacement vector (mm)"

== system Copy_of_Model_vmaRHTS_R2019b/Subsystem4 ==
  Filtered actuator displacement vector : Inport
  Ground_Acceleration : Inport  Port=2
  " NUMERICAL SUBSTRUCTURE" : Subsystem
      mask Display: image('$imagefile'); % Use "Edit Image" on toolstrip to change.
  Coordinate transformation: Actuator to Frame : Subsystem
  Coordinate transformation: Frame to Actuator : Subsystem
  Feedback Force Computation : Subsystem
  Target actuator displacement vector (mm) : Outport
  wires:
  Coordinate transformation: Actuator to Frame/1("[x, theta] (m, rad)") -> Feedback Force Computation/1("[x_est, theta_est] (m,rad)")
  Filtered actuator displacement vector/1 -> Coordinate transformation: Actuator to Frame/1("[xm1_est, xm2_est] (mm)")
  Feedback Force Computation/3(M(29)_phys (N*m)) -> " NUMERICAL SUBSTRUCTURE"/4(RTHS_feedback_Moment29)  "Moment at Uncontrolled Node"
  " NUMERICAL SUBSTRUCTURE"/1(Linear Displacement 27) -> Coordinate transformation: Frame to Actuator/1("[x, theta]")  "Target displacement vector Frame coordinates (mm, rad)"
  Feedback Force Computation/2(M(21)_phys (N*m)) -> " NUMERICAL SUBSTRUCTURE"/3(RTHS_feedback_Moment21)  "Moment at Controlled Node"
  Feedback Force Computation/1(F(27)_phys (N)) -> " NUMERICAL SUBSTRUCTURE"/2(RTHS_feedback_Force27)  "Feedback Force at Controlled Node"
  Ground_Acceleration/1 -> " NUMERICAL SUBSTRUCTURE"/1(Ground_Acceleration)
  Coordinate transformation: Frame to Actuator/1("[xa1,xa2] mm") -> Target actuator displacement vector (mm)/1  "Target actuator displacement vector (mm)"

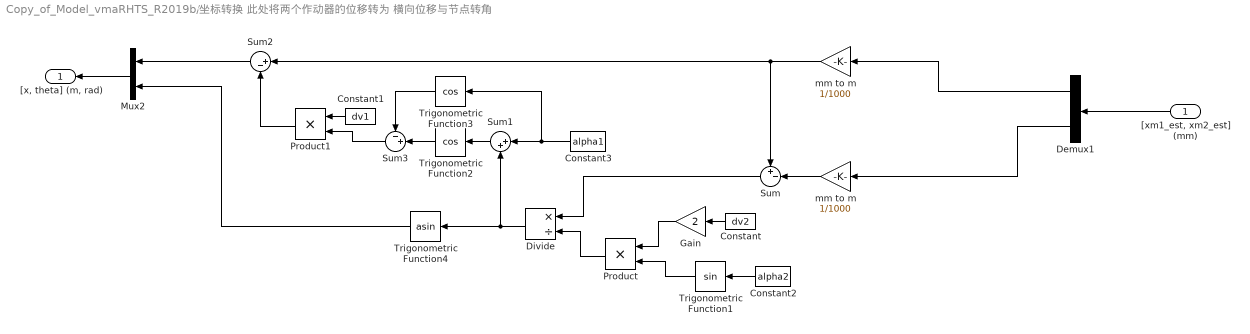
== system Copy_of_Model_vmaRHTS_R2019b/坐标转换 此处将两个作动器的位移转为 横向位移与节点转角  ==
  "[xm1_est, xm2_est] (mm)" : Inport
  Constant : Constant  Value=dv2
  Constant1 : Constant  Value=dv1
  Constant2 : Constant  Value=alpha2
  Constant3 : Constant  Value=alpha1
  Demux1 : Demux  Outputs=2
  Divide : Product  Inputs=*/
  Gain : Gain  Gain=2
  Mux2 : Mux  Inputs=2
  Product : Product
  Product1 : Product
  Sum : Sum  Inputs=+-|
  Sum1 : Sum  Inputs=|++
  Sum2 : Sum  Inputs=|+-
  Sum3 : Sum  Inputs=-+|
  Trigonometric Function1 : Trigonometry
  Trigonometric Function2 : Trigonometry  Operator=cos
  Trigonometric Function3 : Trigonometry  Operator=cos
  Trigonometric Function4 : Trigonometry  Operator=asin
  mm to m : Gain  Gain=1/1000
  "mm to m " : Gain  Gain=1/1000
  "[x, theta] (m, rad)" : Outport  VectorParamsAs1DForOutWhenUnconnected=off
  wires:
  Constant2/1 -> Trigonometric Function1/1
  Constant1/1 -> Product1/1
  Demux1/1 -> mm to m/1
  Demux1/2 -> "mm to m "/1
  Sum/1 -> Divide/1
  Constant/1 -> Gain/1
  Trigonometric Function1/1 -> Product/2
  Gain/1 -> Product/1
  Product/1 -> Divide/2
  Divide/1 -> Sum1/2, Trigonometric Function4/1
  Sum1/1 -> Trigonometric Function2/1
  Constant3/1 -> Sum1/1, Trigonometric Function3/1
  Sum3/1 -> Product1/2
  Sum2/1 -> Mux2/1
  Trigonometric Function2/1 -> Sum3/2
  Trigonometric Function3/1 -> Sum3/1
  Product1/1 -> Sum2/2
  mm to m/1 -> Sum2/1, Sum/1
  "mm to m "/1 -> Sum/2
  Trigonometric Function4/1 -> Mux2/2
  "[xm1_est, xm2_est] (mm)"/1 -> Demux1/1
  Mux2/1 -> "[x, theta] (m, rad)"/1

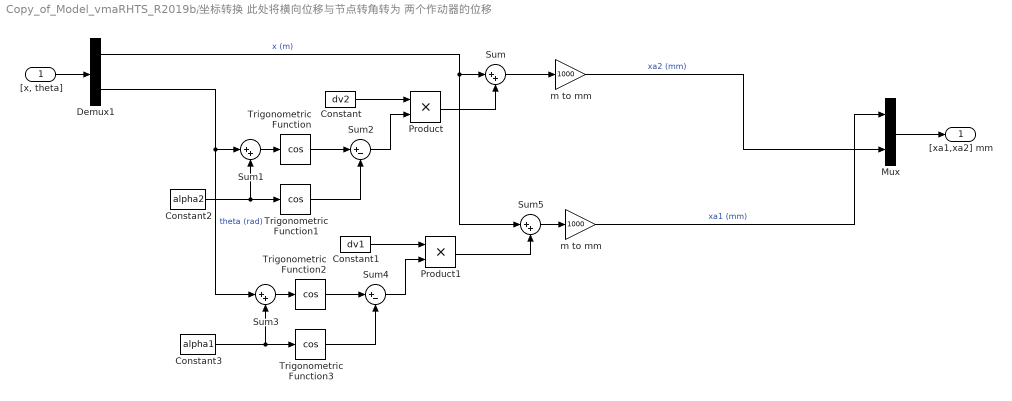
== system Copy_of_Model_vmaRHTS_R2019b/坐标转换 此处将横向位移与节点转角转为 两个作动器的位移 ==
  "[x, theta]" : Inport
  Constant : Constant  Value=dv2
  Constant1 : Constant  Value=dv1
  Constant2 : Constant  Value=alpha2
  Constant3 : Constant  Value=alpha1
  Demux1 : Demux  Outputs=2
  Mux : Mux  Inputs=2
  Product : Product
  Product1 : Product
  Sum{,1,3,5} (4 alike) : Sum  Inputs=|++
  Sum2 : Sum  Inputs=|+-
  Sum4 : Sum  Inputs=|+-
  Trigonometric Function{,1..3} (4 alike) : Trigonometry  Operator=cos
  m to mm : Gain  Gain=1000
  "m to mm " : Gain  Gain=1000
  "[xa1,xa2] mm" : Outport  VectorParamsAs1DForOutWhenUnconnected=off
  wires:
  Constant/1 -> Product/1
  Constant2/1 -> Sum1/2, Trigonometric Function1/1
  Sum1/1 -> Trigonometric Function/1
  Trigonometric Function/1 -> Sum2/1
  Trigonometric Function1/1 -> Sum2/2
  Sum2/1 -> Product/2
  Product/1 -> Sum/2
  Sum/1 -> m to mm/1
  Sum4/1 -> Product1/2
  Trigonometric Function3/1 -> Sum4/2
  Trigonometric Function2/1 -> Sum4/1
  Sum3/1 -> Trigonometric Function2/1
  Constant3/1 -> Sum3/2, Trigonometric Function3/1
  Constant1/1 -> Product1/1
  Product1/1 -> Sum5/2
  Sum5/1 -> "m to mm "/1
  "m to mm "/1 -> Mux/1  "xa1 (mm)"
  m to mm/1 -> Mux/2  "xa2 (mm)"
  Demux1/1 -> Sum/1, Sum5/1  "x (m)"
  "[x, theta]"/1 -> Demux1/1
  Demux1/2 -> Sum3/1, Sum1/1  "theta (rad)"
  Mux/1 -> "[xa1,xa2] mm"/1

== system Copy_of_Model_vmaRHTS_R2019b/控制器与作动器 ==
  Target actuator displacement vector (mm) : Inport
  Control Plant4 : StateSpace  A=A_cplant  B=B_cplant  C=C_cplant  D=D_cplant  InitialCondition=0
  Demux7 : Demux  Outputs=2
  Mux4 : Mux  Inputs=2
  PID Controller2 : slpidlib/PID Controller  Controller=PID  Form=Parallel  TimeDomain=Discrete-time  UseExternalTs=off  SampleTime=-1  IntegratorMethod=Forward Euler  FilterMethod=Forward Euler  ControllerParametersSource=internal  P=1  I=50  UseKiTs=off  D=1e-10  N=100  UseFilter=off  TunerSelectOption=Transfer Function Based (PID Tuner App)  InitialConditionSource=internal  InitialConditionForIntegrator=0  InitialConditionForFilter=0  DifferentiatorICPrevScaledInput=0  ExternalReset=none  TrackingMode=off  Kt=1  LimitOutput=off  SatLimitsSource=internal  UpperSaturationLimit=inf  LowerSaturationLimit=-inf  LinearizeAsGain=on  AntiWindupMode=none  Kb=1  LimitIntegrator=off  UpperIntegratorSaturationLimit=inf  LowerIntegratorSaturationLimit=-inf  POutMin=[]  POutMax=[]  IOutMin=[]  IOutMax=[]  DOutMin=[]  DOutMax=[]  NOutMin=[]  NOutMax=[]  SumOutMin=[]  SumOutMax=[]  SaturationOutMin=[]  SaturationOutMax=[]  PParamMin=[]  PParamMax=[]  IParamMin=[]  IParamMax=[]  DParamMin=[]  DParamMax=[]  NParamMin=[]  NParamMax=[]  KbParamMin=[]  KbParamMax=[]  KtParamMin=[]  KtParamMax=[]  KbOutMin=[]  KbOutMax=[]  KtOutMin=[]  KtOutMax=[]  IntegratorOutMin=[]  IntegratorOutMax=[]  FilterOutMin=[]  FilterOutMax=[]  SumI1OutMin=[]  SumI1OutMax=[]  SumI2OutMin=[]  SumI2OutMax=[]  SumI3OutMin=[]  SumI3OutMax=[]  SumI4OutMin=[]  SumI4OutMax=[]  SumDOutMin=[]  SumDOutMax=[]  DifferentiatorOutMin=[]  DifferentiatorOutMax=[]  FilterDiffOutCoefMin=[]  FilterDiffOutCoefMax=[]  ReciprocalOutMin=[]  ReciprocalOutMax=[]  SumDenOutMin=[]  SumDenOutMax=[]  SumNumOutMin=[]  SumNumOutMax=[]  DivideOutMin=[]  DivideOutMax=[]  UdiffTsProdOutMin=[]  UdiffTsProdOutMax=[]  NTsProdOutMin=[]  NTsProdOutMax=[]  UintegralTsProdOutMin=[]  UintegralTsProdOutMax=[]  UngainTsProdOutMin=[]  UngainTsProdOutMax=[]  ClampingZeroOutDataTypeStr=Inherit: Inherit via back propagation  ClampingZeroOutMin=[]  ClampingZeroOutMax=[]  FilterDenConstantOutDataTypeStr=Inherit: Inherit via back propagation  FilterDenConstantOutMin=[]  FilterDenConstantOutMax=[]  PCopyOutDataTypeStr=Inherit: Inherit via back propagation  PCopyOutMin=[]  PCopyOutMax=[]  NCopyOutDataTypeStr=Inherit: Inherit via back propagation  NCopyOutMin=[]  NCopyOutMax=[]  IntegratorContinuousStateAttributes=''  IntegratorStateMustResolveToSignalObject=off  IntegratorRTWStateStorageClass=Auto  FilterContinuousStateAttributes=''  FilterStateMustResolveToSignalObject=off  FilterRTWStateStorageClass=Auto  ParallelPVariant=InternalParameters  IdealPVariant=Disabled  IVariant=InternalParameters  DVariant=InternalParameters  IntegratorVariant=Discrete  SatVariant=Disabled  AWVariant=Passthrough  PCopyVariant=Disabled  TRVariant=Disabled  FdbkBlocksVariant=Forward  IdealPFdbkVariant=Disabled  SatFdbkVariant=Disabled  DerivativeFilterVariant=Differentiator  NVariant=Passthrough  NCopyVariant=Disabled_SignalSpec  FilterICVariant=InternalICsDifferentiator  IntegratorICVariant=InternalICs  ExternalResetVariant=Disabled  TRSumVariant=Passthrough  SumFdbkVariant=Disabled  SumVariant=Sum_PID  TsampFilterVariant=InternalTs  TsampNgainVariant=Passthrough  TsampIntegralVariant=Disabled_SignalSpec  ExternalSaturationOutDataTypeStr=Inherit: Same as second input
  PID Controller4 : slpidlib/PID Controller  Controller=PID  Form=Parallel  TimeDomain=Discrete-time  UseExternalTs=off  SampleTime=-1  IntegratorMethod=Forward Euler  FilterMethod=Forward Euler  ControllerParametersSource=internal  P=1  I=50  UseKiTs=off  D=1e-10  N=100  UseFilter=on  TunerSelectOption=Transfer Function Based (PID Tuner App)  InitialConditionSource=internal  InitialConditionForIntegrator=0  InitialConditionForFilter=0  DifferentiatorICPrevScaledInput=0  ExternalReset=none  TrackingMode=off  Kt=1  LimitOutput=off  SatLimitsSource=internal  UpperSaturationLimit=inf  LowerSaturationLimit=-inf  LinearizeAsGain=on  AntiWindupMode=none  Kb=1  LimitIntegrator=off  UpperIntegratorSaturationLimit=inf  LowerIntegratorSaturationLimit=-inf  POutMin=[]  POutMax=[]  IOutMin=[]  IOutMax=[]  DOutMin=[]  DOutMax=[]  NOutMin=[]  NOutMax=[]  SumOutMin=[]  SumOutMax=[]  SaturationOutMin=[]  SaturationOutMax=[]  PParamMin=[]  PParamMax=[]  IParamMin=[]  IParamMax=[]  DParamMin=[]  DParamMax=[]  NParamMin=[]  NParamMax=[]  KbParamMin=[]  KbParamMax=[]  KtParamMin=[]  KtParamMax=[]  KbOutMin=[]  KbOutMax=[]  KtOutMin=[]  KtOutMax=[]  IntegratorOutMin=[]  IntegratorOutMax=[]  FilterOutMin=[]  FilterOutMax=[]  SumI1OutMin=[]  SumI1OutMax=[]  SumI2OutMin=[]  SumI2OutMax=[]  SumI3OutMin=[]  SumI3OutMax=[]  SumI4OutMin=[]  SumI4OutMax=[]  SumDOutMin=[]  SumDOutMax=[]  DifferentiatorOutMin=[]  DifferentiatorOutMax=[]  FilterDiffOutCoefMin=[]  FilterDiffOutCoefMax=[]  ReciprocalOutMin=[]  ReciprocalOutMax=[]  SumDenOutMin=[]  SumDenOutMax=[]  SumNumOutMin=[]  SumNumOutMax=[]  DivideOutMin=[]  DivideOutMax=[]  UdiffTsProdOutMin=[]  UdiffTsProdOutMax=[]  NTsProdOutMin=[]  NTsProdOutMax=[]  UintegralTsProdOutMin=[]  UintegralTsProdOutMax=[]  UngainTsProdOutMin=[]  UngainTsProdOutMax=[]  ClampingZeroOutDataTypeStr=Inherit: Inherit via back propagation  ClampingZeroOutMin=[]  ClampingZeroOutMax=[]  FilterDenConstantOutDataTypeStr=Inherit: Inherit via back propagation  FilterDenConstantOutMin=[]  FilterDenConstantOutMax=[]  PCopyOutDataTypeStr=Inherit: Inherit via back propagation  PCopyOutMin=[]  PCopyOutMax=[]  NCopyOutDataTypeStr=Inherit: Inherit via back propagation  NCopyOutMin=[]  NCopyOutMax=[]  IntegratorContinuousStateAttributes=''  IntegratorStateMustResolveToSignalObject=off  IntegratorRTWStateStorageClass=Auto  FilterContinuousStateAttributes=''  FilterStateMustResolveToSignalObject=off  FilterRTWStateStorageClass=Auto  ParallelPVariant=InternalParameters  IdealPVariant=Disabled  IVariant=InternalParameters  DVariant=InternalParameters  IntegratorVariant=Discrete  SatVariant=Disabled  AWVariant=Passthrough  PCopyVariant=Disabled  TRVariant=Disabled  FdbkBlocksVariant=Forward  IdealPFdbkVariant=Disabled  SatFdbkVariant=Disabled  DerivativeFilterVariant=ForwardEulerFilter  NVariant=InternalParameters  NCopyVariant=Disabled  FilterICVariant=InternalICsFilter  IntegratorICVariant=InternalICs  ExternalResetVariant=Disabled  TRSumVariant=Passthrough  SumFdbkVariant=Disabled  SumVariant=Sum_PID  TsampFilterVariant=InternalTs  TsampNgainVariant=Passthrough  TsampIntegralVariant=Disabled_SignalSpec  ExternalSaturationOutDataTypeStr=Inherit: Same as second input
  Sum11 : Sum  Inputs=|+-
  Filtered actuator displacement vector : Outport
  wires:
  PID Controller4/1 -> Mux4/2
  Control Plant4/1 -> Filtered actuator displacement vector/1, Sum11/2  "Filtered actuator displacement vector"
  Demux7/1 -> PID Controller2/1
  Sum11/1 -> Demux7/1
  PID Controller2/1 -> Mux4/1
  Mux4/1 -> Control Plant4/1
  Demux7/2 -> PID Controller4/1
  Target actuator displacement vector (mm)/1 -> Sum11/1

== system Copy_of_Model_vmaRHTS_R2019b/ /Ground motion record ==
  From File : FromFile  FileName=ElCentroAccelNoScaling.mat  SampleTime=dt
  From File1 : FromFile  FileName=KobeAccelNoScaling.mat  SampleTime=dt
  From File2 : FromFile  FileName=MorganAccelNoScaling.mat  SampleTime=dt
  El Centro : Outport
  Kobe : Outport  Port=2
  Morgan : Outport  Port=3
  wires:
  From File/1 -> El Centro/1
  From File2/1 -> Morgan/1
  From File1/1 -> Kobe/1

== system Copy_of_Model_vmaRHTS_R2019b/ 1/Ground motion record ==
  From File : FromFile  FileName=ElCentroAccelNoScaling.mat  SampleTime=dt
  From File1 : FromFile  FileName=KobeAccelNoScaling.mat  SampleTime=dt
  From File2 : FromFile  FileName=MorganAccelNoScaling.mat  SampleTime=dt
  El Centro : Outport
  Kobe : Outport  Port=2
  Morgan : Outport  Port=3
  wires:
  From File/1 -> El Centro/1
  From File2/1 -> Morgan/1
  From File1/1 -> Kobe/1
